simulink model "MotorDC"  (R2013a)
settings: Solver=ode45  StartTime=0.0  StopTime=100.0  RelTol=1e-3
values from neighbouring files (symbols this model uses):
  Den = [(La*Jm) ((Ra*Jm)+(Bm*La)) ((Ra*Bm)+(ki*kv))]    [MotorDCproy3.m]
  Num = [ki]    [MotorDCproy3.m]
settings Model: Creator=user  LastModifiedBy=user

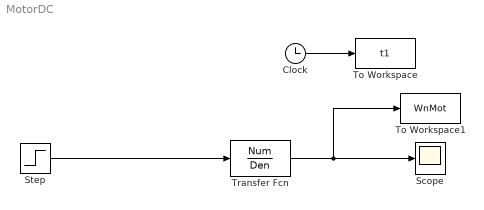
== system MotorDC ==
  Clock : Clock
  Scope : Scope
      settings: YMin=1.0545  YMax=1.0595
  Step : Step  Time=0  After=2  SampleTime=0
  To Workspace : ToWorkspace  VariableName=t1  SampleTime=-1
  To Workspace1 : ToWorkspace  VariableName=WnMot
  Transfer Fcn : TransferFcn  Numerator=Num  Denominator=Den
  wires:
  Step/1 -> Transfer Fcn/1
  Transfer Fcn/1 -> To Workspace1/1, Scope/1
  Clock/1 -> To Workspace/1
